simulink model "chap2_4sim2015b"  (R2015b)
settings: Solver=ode3  StartTime=0.0  StopTime=RunTime  FixedStep=0.01  RelTol=1e-3
settings Model: Creator=Masoud  LastModifiedBy=IT
settings DataIOCC: SaveFormat=Array
settings DebuggingCC: AlgebraicLoopMsg=none  ArtificialAlgebraicLoopMsg=none  InheritedTsInSrcMsg=none  AllowSymbolicDim=on
settings HardwareCC: ProdBitPerPointer=32  ProdLargestAtomicFloat=None  ProdIntDivRoundTo=Undefined  ProdEndianess=Unspecified  ProdWordSize=32  ProdHWDeviceType=32-bit Generic
settings GRTTargetCC: GeneratePreprocessorConditionals=Disable all
settings ConfigComp: CovModelRefEnable=Off

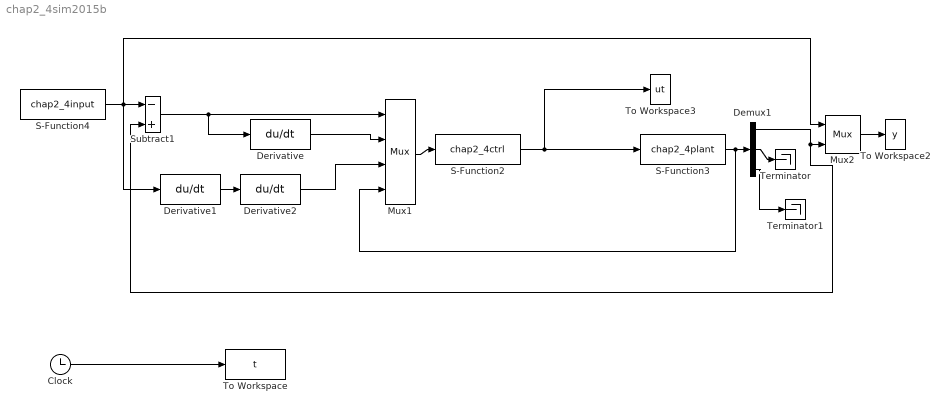
== system chap2_4sim2015b ==
  Clock : Clock
  Demux1 : Demux  Outputs=3
  Derivative : Derivative
  Derivative1 : Derivative
  Derivative2 : Derivative
  Mux1 : Mux
  Mux2 : Mux  Inputs=2
  S-Function2 : S-Function  FunctionName=chap2_4ctrl  SFunctionModules='chap2_4ctrl'  SFunctionDeploymentMode=off  EnableBusSupport=off
  S-Function3 : S-Function  FunctionName=chap2_4plant  SFunctionModules='chap2_4plant'  SFunctionDeploymentMode=off  EnableBusSupport=off
  S-Function4 : S-Function  FunctionName=chap2_4input  SFunctionModules='chap2_4input'  SFunctionDeploymentMode=off  EnableBusSupport=off
  Subtract1 : Sum  Inputs=-+
  Terminator : Terminator
  Terminator1 : Terminator
  To Workspace : ToWorkspace  VariableName=t  SampleTime=-1
  To Workspace2 : ToWorkspace  VariableName=y  SampleTime=-1
  To Workspace3 : ToWorkspace  VariableName=ut  SampleTime=-1
  wires:
  Mux2/1 -> To Workspace2/1
  Demux1/2 -> Terminator/1
  Demux1/3 -> Terminator1/1
  Mux1/1 -> S-Function2/1
  S-Function3/1 -> Mux1/4, Demux1/1
  Demux1/1 -> Subtract1/2, Mux2/2
  Clock/1 -> To Workspace/1
  S-Function2/1 -> S-Function3/1, To Workspace3/1
  S-Function4/1 -> Derivative1/1, Mux2/1, Subtract1/1
  Subtract1/1 -> Derivative/1, Mux1/1
  Derivative/1 -> Mux1/2
  Derivative1/1 -> Derivative2/1
  Derivative2/1 -> Mux1/3
